simulink model "missile_gnc_sim"  (R2025a)
settings: Solver=ode45  StartTime=0.0  StopTime=50  RelTol=1e-3
model workspace (MAT data in the model file):
  A = Simulink.Parameter
  A.Value = [-1.064  1; 290.26  0]
  A.Complexity = 'real'
  A.Dimensions = [2 2]
  A.DataType = 'auto'
values from neighbouring files (symbols this model uses):
  A = [-1.064, 1.000; 290.26, 0.00]    [missile_gnc.m]
  B = [-0.25; -331.40]    [missile_gnc.m]
  C = [-123.34, 0.00; 0.00, 1.00]    [missile_gnc.m]
  D = [-13.41; 0.00]    [missile_gnc.m]
  dT1 = 0.75    [missile_gnc.m]
  dT2 = 0.25    [missile_gnc.m]
  ELEV_INIT = 10000    [missile_gnc.m]
  ELEV_TARGET = 795    [missile_gnc.m]
  LAT_INIT = 34.2329    [missile_gnc.m]
  LAT_OBS = 34.61916    [missile_gnc.m]
  LAT_TARGET = 34.6588    [missile_gnc.m]
  LON_INIT = -119.4573    [missile_gnc.m]
  LON_OBS = -118.8429    [missile_gnc.m]
  LON_TARGET = -118.769745    [missile_gnc.m]
  vel = 1021.08    [missile_gnc.m]
undefined symbols (not defined in the file or in its folder): K, L
libraries: simulink x3, slpidlib x1
settings Model: Creator=naitik  LastModifiedBy=naitik

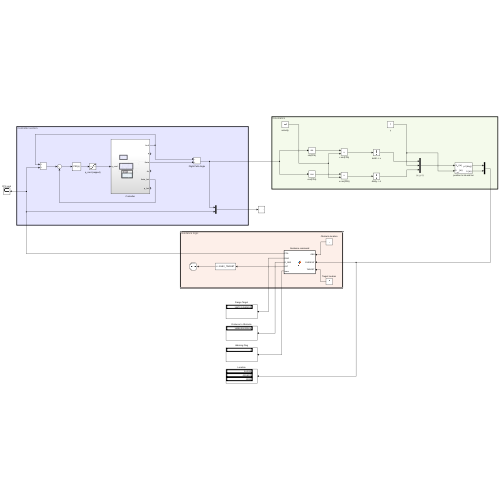
[thumbnail: Simulink's stored preview of the top-level diagram]
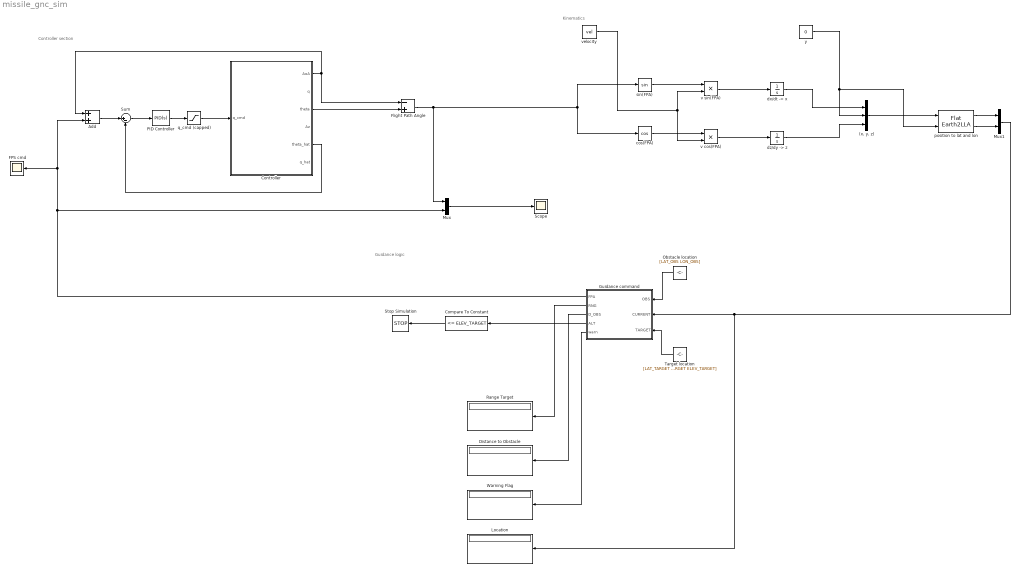
== system missile_gnc_sim ==
  note: Guidance logic
  note: Kinematics
  note: Controller section
  "(x, y, z)" : Mux  Inputs=3
  Add : Sum
  Compare To Constant : simulink/Logic and Bit Operations/Compare To Constant  relop=<=  const=ELEV_TARGET  OutDataTypeStr=boolean
  Controller : Subsystem
  Distance to Obstacle : Display
  FPS cmd : Scope
      settings: ActiveDisplayYMinimum=-0.25022168876961703  ActiveDisplayYMaximum=0.39034798703520079  DataLoggingVariableName=ScopeData8
  Flight Path Angle : Sum  Inputs=-+
  Guidance command : MATLAB Function  TreatAsAtomicUnit=on
  Location : Display
  Mux : Mux  Inputs=2
  Mux1 : Mux  Inputs=2
  Obstacle location : Constant  Value=[LAT_OBS LON_OBS]
  PID Controller : slpidlib/PID Controller  Controller=PID  Form=Parallel  TimeDomain=Continuous-time  UseExternalTs=off  SampleTime=-1  IntegratorMethod=Forward Euler  FilterMethod=Forward Euler  ControllerParametersSource=internal  P=-1  I=0  UseKiTs=off  D=0  UseExternalDerivativeSource=off  N=100  UseFilter=on  TunerSelectOption=Transfer Function Based (PID Tuner App)  InitialConditionSource=internal  InitialConditionForIntegrator=0  InitialConditionForFilter=0  DifferentiatorICPrevScaledInput=0  ExternalReset=none  TrackingMode=off  Kt=1  LimitOutput=off  SatLimitsSource=internal  UpperSaturationLimit=inf  LowerSaturationLimit=-inf  LinearizeAsGain=on  AntiWindupMode=none  Kb=1  LimitIntegrator=off  UpperIntegratorSaturationLimit=inf  LowerIntegratorSaturationLimit=-inf  POutMin=[]  POutMax=[]  IOutMin=[]  IOutMax=[]  DOutMin=[]  DOutMax=[]  NOutMin=[]  NOutMax=[]  SumOutMin=[]  SumOutMax=[]  SaturationOutMin=[]  SaturationOutMax=[]  PParamMin=[]  PParamMax=[]  IParamMin=[]  IParamMax=[]  DParamMin=[]  DParamMax=[]  NParamMin=[]  NParamMax=[]  KbParamMin=[]  KbParamMax=[]  KtParamMin=[]  KtParamMax=[]  KbOutMin=[]  KbOutMax=[]  KtOutMin=[]  KtOutMax=[]  IntegratorOutMin=[]  IntegratorOutMax=[]  FilterOutMin=[]  FilterOutMax=[]  SumI1OutMin=[]  SumI1OutMax=[]  SumI2OutMin=[]  SumI2OutMax=[]  SumI3OutMin=[]  SumI3OutMax=[]  SumI4OutMin=[]  SumI4OutMax=[]  SumDOutMin=[]  SumDOutMax=[]  DifferentiatorOutMin=[]  DifferentiatorOutMax=[]  FilterDiffOutCoefMin=[]  FilterDiffOutCoefMax=[]  ReciprocalOutMin=[]  ReciprocalOutMax=[]  SumDenOutMin=[]  SumDenOutMax=[]  SumNumOutMin=[]  SumNumOutMax=[]  DivideOutMin=[]  DivideOutMax=[]  UdiffTsProdOutMin=[]  UdiffTsProdOutMax=[]  NTsProdOutMin=[]  NTsProdOutMax=[]  UintegralTsProdOutMin=[]  UintegralTsProdOutMax=[]  UngainTsProdOutMin=[]  UngainTsProdOutMax=[]  ClampingZeroOutDataTypeStr=Inherit: Inherit via back propagation  ClampingZeroOutMin=[]  ClampingZeroOutMax=[]  FilterDenConstantOutDataTypeStr=Inherit: Inherit via back propagation  FilterDenConstantOutMin=[]  FilterDenConstantOutMax=[]  PCopyOutDataTypeStr=Inherit: Inherit via back propagation  PCopyOutMin=[]  PCopyOutMax=[]  NCopyOutDataTypeStr=Inherit: Inherit via back propagation  NCopyOutMin=[]  NCopyOutMax=[]  IntegratorContinuousStateAttributes=''  IntegratorStateMustResolveToSignalObject=off  IntegratorRTWStateStorageClass=Auto  FilterContinuousStateAttributes=''  FilterStateMustResolveToSignalObject=off  FilterRTWStateStorageClass=Auto  ParallelPVariant=InternalParameters  IdealPVariant=Disabled  IVariant=InternalParameters  DVariant=InternalParameters  IntegratorVariant=Continuous  SatVariant=Disabled  AWVariant=Passthrough  PCopyVariant=Disabled  TRVariant=Disabled  FdbkBlocksVariant=Forward  IdealPFdbkVariant=Disabled  SatFdbkVariant=Disabled  DerivativeFilterVariant=ContFilter  NVariant=InternalParameters  NCopyVariant=Disabled  FilterICVariant=InternalICsFilter  IntegratorICVariant=InternalICs  ExternalResetVariant=Disabled  TRSumVariant=Passthrough  SumFdbkVariant=Disabled  SumVariant=Sum_PID  TsampFilterVariant=InternalTs  TsampNgainVariant=Passthrough  TsampIntegralVariant=Disabled_SignalSpec  ExternalSaturationOutDataTypeStr=Inherit: Same as second input  DerivativeSourceVariant=ErrorSignal  PreIntVariant=InternalPreInt
  Range Target : Display
  Scope : Scope
      settings: ActiveDisplayYMinimum=-7.5060749138761436  ActiveDisplayYMaximum=6.9571217250321036
  Stop Simulation : Stop
  Sum : Sum  Inputs=|+-
  Target location : Constant  Value=[LAT_TARGET LON_TARGET ELEV_TARGET]
  Warning Flag : Display
  cos(FPA) : Trigonometry  Operator=cos
  "dx/dt -> x" : Integrator
  "dz/dy -> z" : Integrator  InitialCondition=-ELEV_INIT
  position to lat and lon : FlatEarth2LLA  LL0=[LAT_INIT LON_INIT]  psi=yaw_init
  q_cmd (capped) : Saturate  UpperLimit=1  LowerLimit=-1
  sin(FPA) : Trigonometry
  v cos(FPA) : Product
  v sin(FPA) : Product
  velocity : Constant  Value=vel
  y : Constant  Value=0
  wires:
  PID Controller/1 -> q_cmd (capped)/1
  q_cmd (capped)/1 -> Controller/1(q_cmd)
  Controller/5(theta_hat) -> Sum/2
  Sum/1 -> PID Controller/1
  Add/1 -> Sum/1
  Controller/3(theta) -> Flight Path Angle/2
  Controller/1(AoA) -> Add/1, Flight Path Angle/1
  Mux/1 -> Scope/1
  Flight Path Angle/1 -> cos(FPA)/1, sin(FPA)/1, Mux/1
  Guidance command/1(FPA) -> FPS cmd/1, Add/2, Mux/2
  cos(FPA)/1 -> v cos(FPA)/1
  sin(FPA)/1 -> v sin(FPA)/1
  velocity/1 -> v cos(FPA)/2, v sin(FPA)/2
  v sin(FPA)/1 -> "dx/dt -> x"/1
  v cos(FPA)/1 -> "dz/dy -> z"/1
  "dx/dt -> x"/1 -> "(x, y, z)"/1
  "dz/dy -> z"/1 -> "(x, y, z)"/3
  "(x, y, z)"/1 -> position to lat and lon/1
  y/1 -> position to lat and lon/2, "(x, y, z)"/2
  Obstacle location/1 -> Guidance command/1(OBS)
  Target location/1 -> Guidance command/3(TARGET)
  position to lat and lon/1 -> Mux1/1
  position to lat and lon/2 -> Mux1/2
  Compare To Constant/1 -> Stop Simulation/1
  Guidance command/4(ALT) -> Compare To Constant/1
  Mux1/1 -> Location/1, Guidance command/2(CURRENT)
  Guidance command/5(warn) -> Warning Flag/1
  Guidance command/3(D_OBS) -> Distance to Obstacle/1
  Guidance command/2(RNG) -> Range Target/1

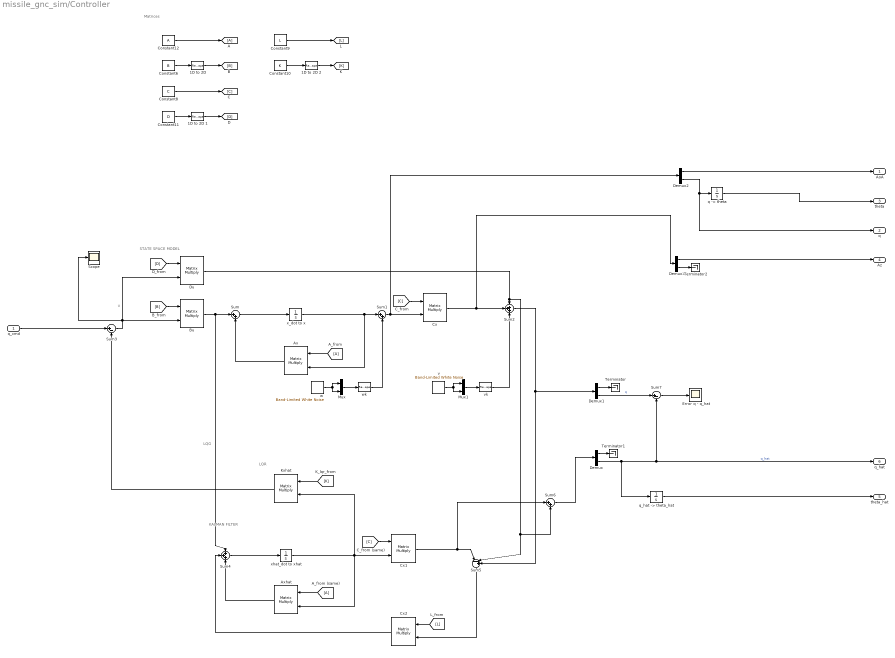
== system missile_gnc_sim/Controller ==
  note: Matrices
  note: LQR
  note: KALMAN FILTER
  note: u
  note: STATE SPACE MODEL
  note: LQG
  q_cmd : Inport
  1D to 2D : Reshape  OutputDimensionality=Customize  OutputDimensions=[2,1]
  1D to 2D 1 : Reshape  OutputDimensionality=Customize  OutputDimensions=[2,1]
  1D to 2D 2 : Reshape  OutputDimensionality=Customize  OutputDimensions=[1,2]
  A : Goto
  A_from : From
  A_from (same) : From
  Ax : Product  Multiplication=Matrix(*)
  Axhat : Product  Multiplication=Matrix(*)
  Bu : Product  Multiplication=Matrix(*)
  Constant10 : Constant  Value=K
  Constant11 : Constant  Value=D
  Constant12 : Constant  Value=A
  Constant6 : Constant  Value=B
  Constant8 : Constant  Value=C
  Constant9 : Constant  Value=L
  Cx : Product  Multiplication=Matrix(*)
  Cx1 : Product  Multiplication=Matrix(*)
  Cx2 : Product  Multiplication=Matrix(*)
  Demux{,1..3} (4 alike) : Demux  Outputs=2
  Du : Product  Multiplication=Matrix(*)
  Error q - q_hat : Scope
      settings: ActiveDisplayYMinimum=-25.414241575358218  ActiveDisplayYMaximum=28.894514030750905  DataLoggingVariableName=ScopeData2
  Kxhat : Product  Multiplication=Matrix(*)
  Mux : Mux  Inputs=2
  Mux1 : Mux  Inputs=2
  Scope : Scope
      settings: ActiveDisplayYMinimum=-18.884376695520043  ActiveDisplayYMaximum=23.948070292052293
  Sum : Sum  Inputs=|++
  Sum1 : Sum  Inputs=|++
  Sum2 : Sum  Inputs=+++
  Sum3 : Sum  Inputs=|+-
  Sum4 : Sum  Inputs=+++
  Sum5 : Sum  Inputs=|--+
  Sum6 : Sum  Inputs=|++
  Sum7 : Sum  Inputs=|+-
  Terminator : Terminator
  Terminator1 : Terminator
  Terminator2 : Terminator
  "q -> theta" : Integrator
  "q_hat -> theta_hat" : Integrator
  v : simulink/Sources/Band-Limited White Noise  Cov=[0.00001]  Ts=dT2  seed=[23341]
  vk : Reshape  OutputDimensionality=Column vector (2-D)
  w : simulink/Sources/Band-Limited White Noise  Cov=0.00000001  Ts=dT1  seed=[23341]
  wk : Reshape  OutputDimensionality=Column vector (2-D)
  x_dot to x : Integrator
  xhat_dot to xhat : Integrator
  AoA : Outport
  q : Outport  Port=2
  theta : Outport  Port=3
  Az : Outport  Port=4
  theta_hat : Outport  Port=5
  q_hat : Outport  Port=6
  wires:
  Constant6/1 -> 1D to 2D/1
  1D to 2D 2/1 -> [K]
  1D to 2D/1 -> [B]
  Constant8/1 -> [C]
  Constant10/1 -> 1D to 2D 2/1
  Constant9/1 -> [L]
  Constant11/1 -> 1D to 2D 1/1
  Constant12/1 -> A/1
  1D to 2D 1/1 -> [D]
  Bu/1 -> Sum/1, Sum4/1
  Sum7/1 -> Error q - q_hat/1
  Demux3/1 -> Az/1
  "q_hat -> theta_hat"/1 -> theta_hat/1
  Demux2/2 -> q/1, "q -> theta"/1
  [B] -> Bu/1
  [L] -> Cx2/1
  Sum3/1 -> Scope/1, Bu/2, Du/2
  Sum6/1 -> Demux/1
  Sum4/1 -> xhat_dot to xhat/1
  Demux1/1 -> Terminator/1
  Axhat/1 -> Sum4/3
  Demux/2 -> "q_hat -> theta_hat"/1, q_hat/1, Sum7/2  "q_hat"
  [D] -> Du/1
  [C] -> Cx/1
  Sum/1 -> x_dot to x/1
  x_dot to x/1 -> Ax/2, Sum1/1
  xhat_dot to xhat/1 -> Axhat/2, Kxhat/2, Cx1/2
  Sum5/1 -> Cx2/2
  w/1 -> Mux/1, Mux/2
  "q -> theta"/1 -> theta/1
  Cx1/1 -> Sum6/1, Sum5/1
  A_from (same)/1 -> Axhat/1
  Sum1/1 -> Demux2/1, Cx/2
  Cx2/1 -> Sum4/2
  Demux1/2 -> Sum7/1  "q"
  [K] -> Kxhat/1
  Cx/1 -> Demux3/1, Sum2/2
  Ax/1 -> Sum/2
  Sum2/1 -> Demux1/1, Sum5/3
  Demux3/2 -> Terminator2/1
  A_from/1 -> Ax/1
  [C] -> Cx1/1
  Demux/1 -> Terminator1/1
  vk/1 -> Sum2/3
  Kxhat/1 -> Sum3/2
  Du/1 -> Sum6/2, Sum5/2, Sum2/1
  wk/1 -> Sum1/2
  Demux2/1 -> AoA/1
  Mux/1 -> wk/1
  q_cmd/1 -> Sum3/1
  v/1 -> Mux1/1, Mux1/2
  Mux1/1 -> vk/1

== matlab function missile_gnc_sim/Guidance command ==
  data: OBS input; FPA output; CURRENT input; TARGET input; RNG output; D_OBS output; ALT output; warn output
function [FPA, RNG, D_OBS, ALT, warn] = fcn(OBS, CURRENT, TARGET)
%#codegen

R = 6.371e3;
d2r = pi/180;

%OBSTACLE LOCATION
LAT_OBS = OBS(1);
LON_OBS = OBS(2);

%OBSTACLE THRESHOLD (NO GO ZONE)
thres = 2000;

%TARGET LOCATION
LAT_TARGET = TARGET(1);
LON_TARGET = TARGET(2);
ELEV_TARGET = TARGET(3);

%CURRENT LOCATION
ELEV_CUR = CURRENT(1);
LAT_CUR = CURRENT(2);
LON_CUR = CURRENT(3);

%% DISTANCE TO TARGET
l1 = LAT_CUR * d2r;
u1 = LON_CUR * d2r;
l2 = LAT_TARGET  * d2r;
u2 = LON_TARGET  * d2r;

dl = l2 - l1;
du = u2 - u1;

% Haversine formula
a = sin(dl/2)^2 + cos(l1)*cos(l2)*sin(du/2)^2;
c = 2 * atan2(sqrt(a), sqrt(1 - a));
d = R * c;
%% DISTANCE FROM OBSTACLE
l3 = LAT_OBS  * d2r;
u3 = LON_OBS  * d2r;

dh = abs(ELEV_TARGET - ELEV_CUR);

dl = l3 - l1;
du = u3 - u1;

% Haversine formula
a = sin(dl/2)^2 + cos(l1)*cos(l2)*sin(du/2)^2;
c = 2 * atan2(sqrt(a), sqrt(1 - a));
d_obs = R * c;
%% CURRENT RANGE (FROM TARGATE) - RANGE > DISTANCE
range = sqrt(d^2 + dh^2);
%% CALCULATE COMMAND FLIGHT PATH SETPOINT BASED ON d_obs, range
if abs(d_obs) >= thres
    w = 0;
    FPA_CMD = atan(dh/d);
else
    w = 1;
    FPA_CMD = 0;
end


%% OUTPUT VARIABLES

FPA = FPA_CMD;
RNG = range;
D_OBS = d_obs;
warn = w;
ALT = ELEV_CUR;
